simulink model "wheelset_KALKER"  (Simulink 7.8)
settings: Solver=FixedStepDiscrete  StartTime=0.0  StopTime=10.0  FixedStep=Delta_t  RelTol=1e-3
undefined symbols (not defined in the file or in its folder): Delta_t
settings Model: Creator=imac  LastModifiedBy=aitor
settings DebuggingCC: FcnCallInpInsideContextMsg=Use local settings

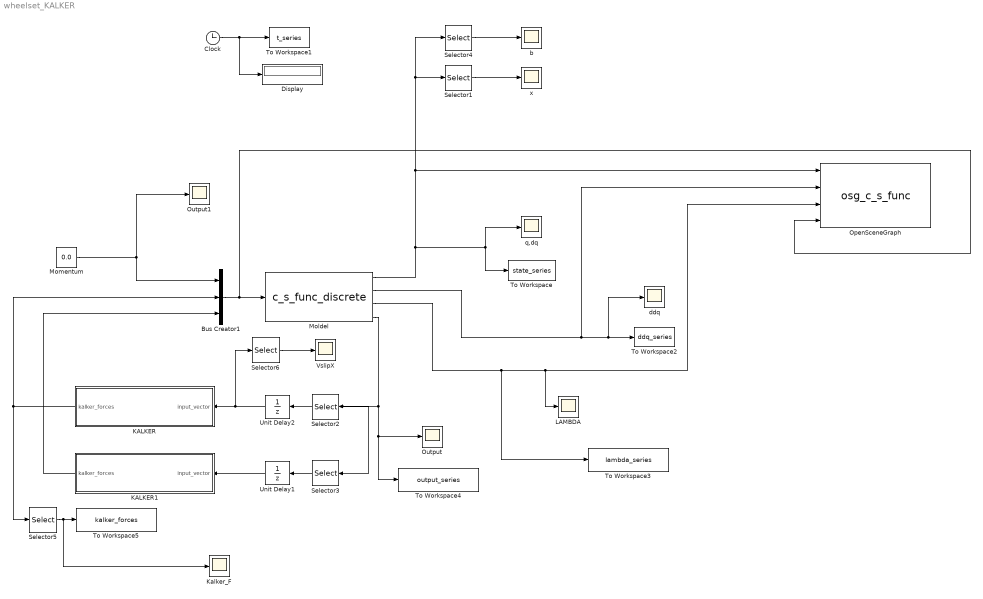
== system wheelset_KALKER ==
  " b" : Scope
      settings: YMin=0.205  YMax=0.22  SaveName=ScopeData4  SampleInput=on
  Bus Creator1 : BusCreator  Inputs=3
  Clock : Clock
  Display : Display
  KALKER : MATLAB Function  TreatAsAtomicUnit=on  SystemSampleTime=Delta_t
  KALKER1 : MATLAB Function  TreatAsAtomicUnit=on  SystemSampleTime=Delta_t
  Kalker_F : Scope
      settings: TimeRange=0.007457627118644068  YMin=-123.556  YMax=-123.556  SaveName=ScopeData7  SampleInput=on
  LAMBDA : Scope
      settings: YMin=-1  YMax=6  SaveName=ScopeData2  SampleInput=on
  Moldel : S-Function  FunctionName=c_s_func_discrete  Parameters=q dq param Delta_t  EnableBusSupport=off
      mask Type: S-function: mycsfunc
      mask Description: This is a S-function that does the continuous state space system.
      mask Display: disp('[M , Phi_q''] [ddq]\n[Phi_q , 0] [lambda]\n=\n [Q ] \n   [gamma] ');
  Momentum : Constant  Value=0.0
  OpenSceneGraph : S-Function  FunctionName=osg_c_s_func  Parameters=param  EnableBusSupport=off
  Output : Scope
      settings: YMin=0  YMax=1.4e-16  SaveName=ScopeData3  SampleInput=on
  Output1 : Scope
      settings: YMin=0  YMax=1.4e-16  SaveName=ScopeData8  SampleInput=on
  Selector1 : Selector  InputPortWidth=28  IndexOptions=Index vector (dialog)  Indices=1  OutputSizes=1
  Selector2 : Selector  InputPortWidth=16  IndexOptions=Index vector (dialog)  Indices=1:1:8  OutputSizes=1
  Selector3 : Selector  InputPortWidth=16  IndexOptions=Index vector (dialog)  Indices=9:1:16  OutputSizes=1
  Selector4 : Selector  InputPortWidth=28  IndexOptions=Index vector (dialog)  Indices=5  OutputSizes=1
  Selector5 : Selector  InputPortWidth=3  IndexOptions=Index vector (dialog)  Indices=1  OutputSizes=1
  Selector6 : Selector  InputPortWidth=8  IndexOptions=Index vector (dialog)  Indices=2  OutputSizes=1
  To Workspace : ToWorkspace  VariableName=state_series  SampleTime=-1  SaveFormat=Array
  To Workspace1 : ToWorkspace  VariableName=t_series  SampleTime=-1  SaveFormat=Array
  To Workspace2 : ToWorkspace  VariableName=ddq_series  SampleTime=-1  SaveFormat=Array
  To Workspace3 : ToWorkspace  VariableName=lambda_series  SampleTime=-1  SaveFormat=Array
  To Workspace4 : ToWorkspace  VariableName=output_series  SampleTime=-1  SaveFormat=Array
  To Workspace5 : ToWorkspace  VariableName=kalker_forces  SampleTime=-1  SaveFormat=Array
  Unit Delay1 : UnitDelay  SampleTime=-1
  Unit Delay2 : UnitDelay  SampleTime=-1
  VslipX : Scope
      settings: YMin=0.054  YMax=0.0605  SaveName=ScopeData6  SampleInput=on
  ddq : Scope
      settings: YMin=-500  YMax=300  SampleInput=on
  q,dq : Scope
      settings: YMin=-0.03  YMax=0.17  SampleInput=on
  x : Scope
      settings: TimeRange=0.15  YMin=0.3085  YMax=0.3165  SaveName=ScopeData5  SampleInput=on
  wires:
  Clock/1 -> To Workspace1/1, Display/1
  Moldel/1 -> q,dq/1, To Workspace/1, OpenSceneGraph/1, Selector1/1, Selector4/1
  Moldel/2 -> OpenSceneGraph/2, ddq/1, To Workspace2/1
  Moldel/3 -> To Workspace3/1, LAMBDA/1, OpenSceneGraph/3
  Moldel/4 -> Selector2/1, Selector3/1, Output/1, To Workspace4/1
  Momentum/1 -> Bus Creator1/1, Output1/1
  Bus Creator1/1 -> Moldel/1, OpenSceneGraph/4
  Unit Delay2/1 -> Selector6/1, KALKER/1(input_vector)
  Unit Delay1/1 -> KALKER1/1(input_vector)
  Selector1/1 -> x/1
  Selector4/1 -> " b"/1
  Selector6/1 -> VslipX/1
  Selector5/1 -> To Workspace5/1, Kalker_F/1
  KALKER1/1(kalker_forces) -> Bus Creator1/3
  KALKER/1(kalker_forces) -> Selector5/1, Bus Creator1/2
  Selector3/1 -> Unit Delay1/1
  Selector2/1 -> Unit Delay2/1

== matlab function KALKER1 ==
  data: input_vector input double; kalker_forces output double
function kalker_forces = fcn(input_vector)
%#codegen
coder.extrinsic('kalker_coeff','Hertz_ellipse','Kalker_linear'); 


N = input_vector(1);
Vxslip = input_vector(2);
Vyslip = input_vector(3);
OMzslip = input_vector(4);
Omega = input_vector(5);
Vo = input_vector(6);
R = input_vector(7);
r = input_vector(8);


E = 210e9; % MPa
nu = 0.27; %Steel
G = E/(2*(1-nu)); % MPa


if R == 0 
    R = 0.5;
end
if r == 0 
    r = 0.1;
end

Ry_w = R; % m
Rx_r = r; % m 
Ry_r = inf; % m
Rx_w = inf; % m  
Radii = [Rx_w,Rx_r,Ry_w,Ry_r];


[a,b] = Hertz_ellipse(N,Radii,E,nu);

%KalkerCoeff = kalker_coeff(a,b,nu);
if sqrt(Vxslip^2 + Vyslip^2 + OMzslip^2 ) > 1e-8
  %Vx  = (Vxslip - R*Omega) / (abs(0.5 * (Vxslip + R*Omega) )); %javier
  Vx  = (Vo - R*Omega) / (abs(0.5 * (Vo + R*Omega) ));
  %Vx1  = (Vxslip - Vo) / abs((0.5 * (Vxslip + Vo))) 
  %Vx2  = Vxslip /  abs(Vo)  % Fisette
  if abs(Vx)>=0.04
    Vx=sign(Vx)*0.04;
  end
  Vy  = 0;%Output_(4) / (0.5*Output_(4) + Output_(1));
  Phi = 0;%Output_(5) / (0.5*Output_(5) + Output_(1));
else 
    Vx  = 0;
    Vy  = 0;
    Phi = 0;
end 
Vcreep = [Vx;Vy;Phi];

mu=0.4;
Delta_t=0.001;

kalker_forces = zeros(3,1);
if Vxslip < 9.8*Delta_t && Vo < 0.1%9.8*Delta_t
   kalker_forces(1) = -(mu*N /(Delta_t*9.8))*Vxslip
else    
    kalker_forces = 1*Kalker_linear(Vcreep,a,b,G,nu);
end


if abs(kalker_forces(1))>=N
   kalker_forces(1) = mu*sign(kalker_forces(1))*N;
end

%Fp=sqrt(kalker_forces(1)^2 +kalker_forces(2)^2 );
%if Fp <= 3*mu*N
%    F = mu * N * ( Fp/(mu*N) - (1/3)*(Fp/(mu*N))^2 + (1/27)*(Fp/(mu*N))^3 );
%elseif Fp > 3*mu*N
%    F = mu*N;
%end
%kalker_forces(1) =sign(kalker_forces(1))* Fp;

== matlab function KALKER ==
  data: input_vector input double; kalker_forces output double
function kalker_forces = fcn(input_vector)
%#codegen
coder.extrinsic('kalker_coeff','Hertz_ellipse','Kalker_linear'); 


N = input_vector(1);
Vxslip = input_vector(2);
Vyslip = input_vector(3);
OMzslip = input_vector(4);
Omega = input_vector(5);
Vo = input_vector(6);
R = input_vector(7);
r = input_vector(8);


E = 210e9; % MPa
nu = 0.27; %Steel
G = E/(2*(1-nu)); % MPa


if R == 0 
    R = 0.5;
end
if r == 0 
    r = 0.1;
end

Ry_w = R; % m
Rx_r = r; % m 
Ry_r = inf; % m
Rx_w = inf; % m  
Radii = [Rx_w,Rx_r,Ry_w,Ry_r];


[a,b] = Hertz_ellipse(N,Radii,E,nu);

%KalkerCoeff = kalker_coeff(a,b,nu);
if sqrt(Vxslip^2 + Vyslip^2 + OMzslip^2 ) > 1e-8
  %Vx  = (Vxslip - R*Omega) / (abs(0.5 * (Vxslip + R*Omega) )); %javier
  Vx  = (Vo - R*Omega) / (abs(0.5 * (Vo + R*Omega) ));
  %Vx1  = (Vxslip - Vo) / abs((0.5 * (Vxslip + Vo))) 
  %Vx2  = Vxslip /  abs(Vo)  % Fisette
  if abs(Vx)>=0.04
    Vx=sign(Vx)*0.04;
  end
  Vy  = 0;%Output_(4) / (0.5*Output_(4) + Output_(1));
  Phi = 0;%Output_(5) / (0.5*Output_(5) + Output_(1));
else 
    Vx  = 0;
    Vy  = 0;
    Phi = 0;
end 
Vcreep = [Vx;Vy;Phi];

mu=0.4;
Delta_t=0.001;

kalker_forces = zeros(3,1);
if Vxslip < 9.8*Delta_t && Vo < 0.1%9.8*Delta_t
   kalker_forces(1) = -(mu*N /(Delta_t*9.8))*Vxslip
else    
    kalker_forces = 1*Kalker_linear(Vcreep,a,b,G,nu);
end


if abs(kalker_forces(1))>=N
   kalker_forces(1) = mu*sign(kalker_forces(1))*N;
end

%Fp=sqrt(kalker_forces(1)^2 +kalker_forces(2)^2 );
%if Fp <= 3*mu*N
%    F = mu * N * ( Fp/(mu*N) - (1/3)*(Fp/(mu*N))^2 + (1/27)*(Fp/(mu*N))^3 );
%elseif Fp > 3*mu*N
%    F = mu*N;
%end
%kalker_forces(1) =sign(kalker_forces(1))* Fp;
